simulink model "ysw8_4"  (R2014a)
settings: Solver=ode15s  StartTime=0.0  StopTime=0.2  RelTol=1e-3
libraries: powerlib x9
settings Model: Creator=Administrator  LastModifiedBy=Administrator

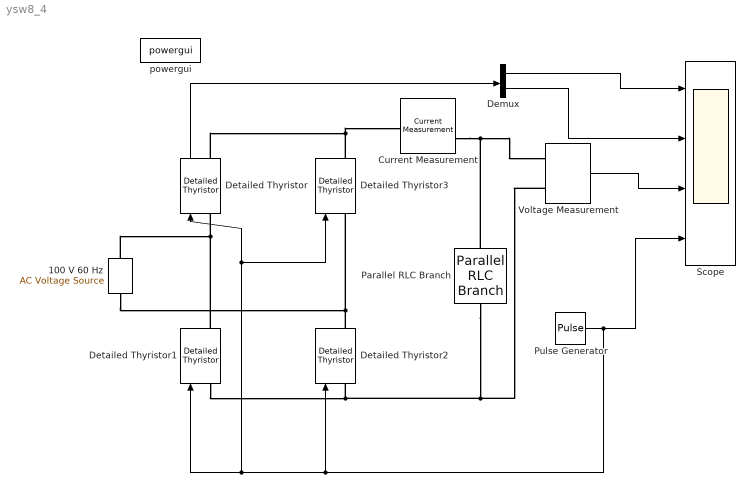
== system ysw8_4 ==
  100 V 60 Hz : powerlib/Electrical Sources/AC Voltage Source  Description=source block  Amplitude=100  Phase=0  Frequency=50  SampleTime=0  Measurements=None
      settings: AttributesFormatString=\n
  Current Measurement : powerlib/Measurements/Current Measurement  PhasorSimulation=off  OutputType=Complex  PSBequivalent=0
  Demux : Demux  Outputs=2
  Detailed Thyristor{,1..3} (4 alike) : powerlib/Power Electronics/Detailed Thyristor  Ron=0.001  Lon=1e-3  Vf=0.8  IL=0.1  Tq=100e-6  IC=0  Rs=500  Cs=250e-9  Measurements=on
  Parallel RLC Branch : powerlib/Elements/Parallel RLC Branch  LConnTagsString=a  RConnTagsString=__new0  BranchType=R  Resistance=1  Inductance=1e-3  SetiL0=off  InitialCurrent=0  Capacitance=1e-6  Setx0=off  InitialVoltage=0  Measurements=None
  Pulse Generator : DiscretePulseGenerator  PulseType=Time based  Period=0.01  PulseWidth=50  PhaseDelay=0.0017
  Scope : Scope  NumInputPorts=4
      settings: YMin=-5~-5~-5~-5  YMax=5~5~5~5
  Voltage Measurement : powerlib/Measurements/Voltage Measurement  PhasorSimulation=off  OutputType=Complex  PSBequivalent=0
  powergui : powerlib/powergui  SimulationMode=Continuous  SolverType=Tustin  SampleTime=0  frequency=60  SPID=off  DisableSnubberDevices=off  DisableRonSwitches=off  DisableVfSwitches=off  SwTol=0  Interpol=off  DisplayEquations=off  Ts=0  methode=off  frequencyindice=50  Pbase=100e6  ErrMax=1e-4  Iterations=50  UnitsV=kV  UnitsW=MW  FunctionMessages=off  echomessages=off  HookPort=off  EnableUseOfTLC=off  x0status=blocks  RestoreLinks=warning  ResistiveCurrentMeasurement=off  Frange=[0:2:500]  Ylog=off  Xlog=on  ShowGrid=off  save=off  variable=ZData  structure=0  ZoomFFT=on  StartTime=0.0  cycles=1  DisplayStyle=1  fundamental=60  FreqAxis=off  MaxFrequency=1000  frequencyindicesteady=1  RmsSteady=1  display=off
  wires:
  Pulse Generator/1 -> Scope/4, Detailed Thyristor2/1, Detailed Thyristor/1, Detailed Thyristor3/1, Detailed Thyristor1/1
  Voltage Measurement/1 -> Scope/3
  Demux/1 -> Scope/1
  Demux/2 -> Scope/2
  Detailed Thyristor/1 -> Demux/1
  connections:
  100 V 60 Hz/RConn1 -- Detailed Thyristor1/RConn1 -- Detailed Thyristor/LConn1
  Detailed Thyristor3/RConn1 -- Detailed Thyristor/RConn1 -- Current Measurement/LConn1
  Detailed Thyristor2/RConn1 -- 100 V 60 Hz/LConn1 -- Detailed Thyristor3/LConn1
  Parallel RLC Branch/RConn1 -- Voltage Measurement/LConn2 -- Detailed Thyristor1/LConn1 -- Detailed Thyristor2/LConn1
  Current Measurement/RConn1 -- Parallel RLC Branch/LConn1 -- Voltage Measurement/LConn1
